simulink model "RocketAirBrake_Simulation"  (R2018b)
settings: Solver=VariableStepAuto  StartTime=0.0  StopTime=30  RelTol=1e-3
undefined symbols (not defined in the file or in its folder): INTAB1, INTAB3, INTAB4
libraries: embdlinuxlib x5, simulink x1
settings Model: Creator=benkl  LastModifiedBy=Alan

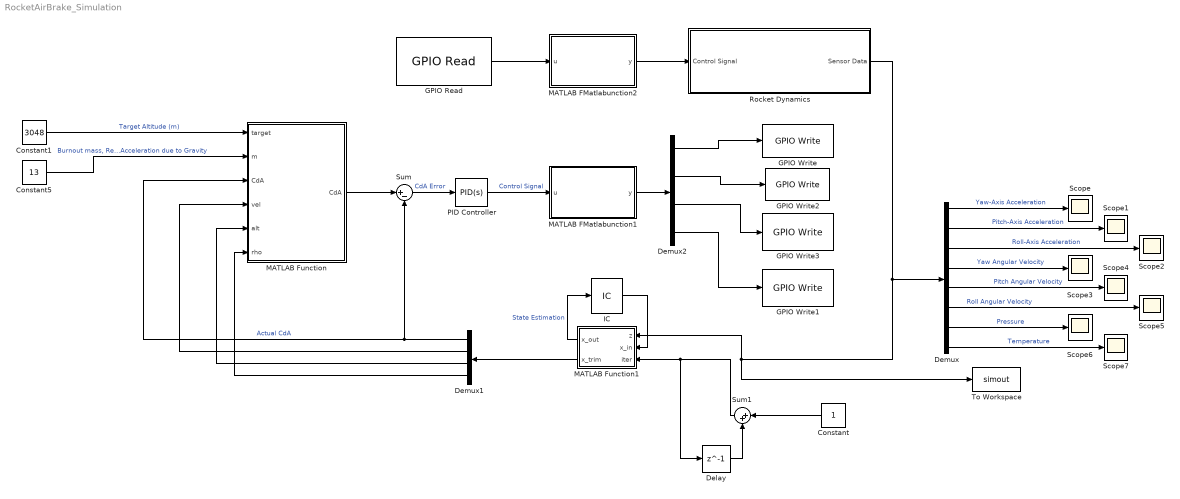
== system RocketAirBrake_Simulation ==
  Constant : Constant
  Constant1 : Constant  Value=3048
  Constant5 : Constant  Value=13
  Delay : Delay  DelayLength=1  InitialCondition=0
  Demux : Demux  Outputs=8
  Demux1 : Demux
  Demux2 : Demux
  GPIO Read : embdlinuxlib/GPIO Read  board=Model B+  gpio=4  internalResistor=Off  sampleTime=0.1  direction=Input  blockPlatform=Raspberry Pi
      settings: SourceProductName=Simulink Support Package for Raspberry Pi Hardware  SourceProductBaseCode=RASPPI
  GPIO Write{,1..3} (4 alike) : embdlinuxlib/GPIO Write  board=Model B+  gpio=17  direction=Output  blockPlatform=Raspberry Pi
      settings: SourceProductName=Simulink Support Package for Raspberry Pi Hardware  SourceProductBaseCode=RASPPI
  IC : InitialCondition  Value=[0;0;0;0;0;0;0;0;0;0;0;0]
  MATLAB FMatlabunction1 : MATLAB Function  TreatAsAtomicUnit=on
  MATLAB FMatlabunction2 : MATLAB Function  TreatAsAtomicUnit=on
  MATLAB Function : MATLAB Function  TreatAsAtomicUnit=on
  MATLAB Function1 : MATLAB Function  TreatAsAtomicUnit=on
  PID Controller : simulink/Continuous/PID Controller  Controller=PID  Form=Parallel  TimeDomain=Continuous-time  SampleTime=-1  IntegratorMethod=Forward Euler  FilterMethod=Forward Euler  ControllerParametersSource=internal  P=1  I=0  D=0  UseFilter=on  N=100  TunerSelectOption=Transfer Function Based (PID Tuner App)  InitialConditionSource=internal  InitialConditionForIntegrator=0  InitialConditionForFilter=0  DifferentiatorICPrevScaledInput=0  ExternalReset=none  TrackingMode=off  Kt=1  LimitOutput=off  UpperSaturationLimit=inf  LowerSaturationLimit=-inf  LinearizeAsGain=on  AntiWindupMode=none  Kb=1  POutMin=[]  POutMax=[]  IOutMin=[]  IOutMax=[]  DOutMin=[]  DOutMax=[]  NOutMin=[]  NOutMax=[]  SumOutMin=[]  SumOutMax=[]  SaturationOutMin=[]  SaturationOutMax=[]  PParamMin=[]  PParamMax=[]  IParamMin=[]  IParamMax=[]  DParamMin=[]  DParamMax=[]  NParamMin=[]  NParamMax=[]  KbParamMin=[]  KbParamMax=[]  KtParamMin=[]  KtParamMax=[]  KbOutMin=[]  KbOutMax=[]  KtOutMin=[]  KtOutMax=[]  IntegratorOutMin=[]  IntegratorOutMax=[]  FilterOutMin=[]  FilterOutMax=[]  SumI1OutMin=[]  SumI1OutMax=[]  SumI2OutMin=[]  SumI2OutMax=[]  SumI3OutMin=[]  SumI3OutMax=[]  SumI4OutMin=[]  SumI4OutMax=[]  SumDOutMin=[]  SumDOutMax=[]  DifferentiatorOutMin=[]  DifferentiatorOutMax=[]  FilterDiffOutCoefMin=[]  FilterDiffOutCoefMax=[]  ReciprocalOutMin=[]  ReciprocalOutMax=[]  SumDenOutMin=[]  SumDenOutMax=[]  SumNumOutMin=[]  SumNumOutMax=[]  DivideOutMin=[]  DivideOutMax=[]  IntegratorContinuousStateAttributes=''  IntegratorStateMustResolveToSignalObject=off  IntegratorRTWStateStorageClass=Auto  FilterContinuousStateAttributes=''  FilterStateMustResolveToSignalObject=off  FilterRTWStateStorageClass=Auto  ParallelPVariant=InternalParameters  IdealPVariant=Disabled  IVariant=InternalParameters  DVariant=InternalParameters  IntegratorVariant=Continuous  SatVariant=Disabled  AWVariant=Passthrough  PCopyVariant=Disabled  TRVariant=Disabled  FdbkBlocksVariant=Forward  IdealPFdbkVariant=Disabled  SatFdbkVariant=Disabled  DerivativeFilterVariant=ContFilter  NVariant=InternalParameters  NCopyVariant=Disabled  FilterICVariant=InternalICsFilter  IntegratorICVariant=InternalICs  ExternalResetVariant=Disabled  TRSumVariant=Passthrough  SumFdbkVariant=Disabled  SumVariant=Sum_PID
  Rocket Dynamics : Subsystem
  Scope{,1..7} (8 alike) : Scope
  Sum : Sum  Inputs=|+-
  Sum1 : Sum  Inputs=|++
  To Workspace : ToWorkspace  VariableName=simout  SaveFormat=Timeseries  SampleTime=-1
  wires:
  Demux/1 -> Scope/1  "Yaw-Axis Acceleration"
  Demux/2 -> Scope1/1  "Pitch-Axis Acceleration"
  Constant1/1 -> MATLAB Function/1(target)  "Target Altitude (m)"
  MATLAB Function/1(CdA) -> Sum/1
  Constant5/1 -> MATLAB Function/2(m)  "Burnout mass, Reference Area,  Acceleration due to Gravity"
  Demux1/1 -> MATLAB Function/3("CdA "), Sum/2  "Actual CdA"
  Demux1/2 -> MATLAB Function/4(vel)
  Demux1/3 -> MATLAB Function/5(alt)
  Demux1/4 -> MATLAB Function/6(rho)
  Sum/1 -> PID Controller/1  "CdA Error"
  Rocket Dynamics/1(Sensor Data) -> To Workspace/1, MATLAB Function1/1(z), Demux/1
  Demux/8 -> Scope7/1  "Temperature"
  Demux/3 -> Scope2/1  "Roll-Axis Acceleration"
  Demux/4 -> Scope3/1  "Yaw Angular Velocity"
  Demux/5 -> Scope4/1  "Pitch Angular Velocity"
  Demux/6 -> Scope5/1  "Roll Angular Velocity"
  Demux/7 -> Scope6/1  "Pressure"
  GPIO Read/1 -> MATLAB FMatlabunction2/1(u)
  MATLAB FMatlabunction2/1(y) -> Rocket Dynamics/1(Control Signal)
  PID Controller/1 -> MATLAB FMatlabunction1/1(u)  "Control Signal"
  MATLAB FMatlabunction1/1(y) -> Demux2/1
  Demux2/4 -> GPIO Write1/1
  Demux2/3 -> GPIO Write3/1
  Demux2/2 -> GPIO Write2/1
  Demux2/1 -> GPIO Write/1
  MATLAB Function1/1(x_out) -> IC/1  "State Estimation"
  MATLAB Function1/2(x_trim) -> Demux1/1
  IC/1 -> MATLAB Function1/2(x_in)
  Constant/1 -> Sum1/1
  Sum1/1 -> Delay/1, MATLAB Function1/3(iter)
  Delay/1 -> Sum1/2

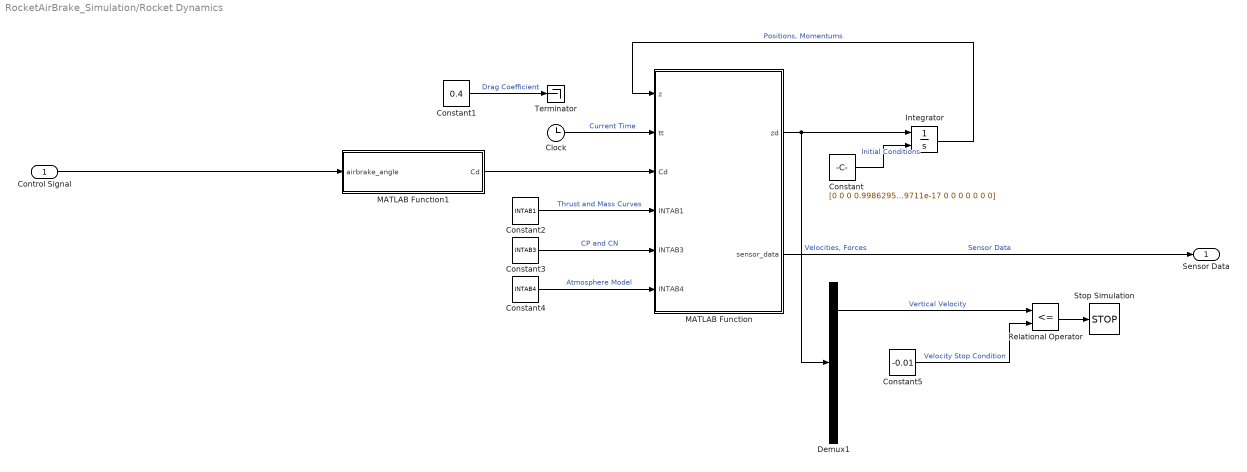
== system RocketAirBrake_Simulation/Rocket Dynamics ==
  Control Signal : Inport
  Clock : Clock
  Constant : Constant  Value="[0\t0\t0\t0.998629534754574\t-0.0523359562429438\t1.92279183879711e-17\t0\t0\t0\t0\t0\t0\t0]"
  Constant1 : Constant  Value=0.4
  Constant2 : Constant  Value=INTAB1  VectorParams1D=off
  Constant3 : Constant  Value=INTAB3  VectorParams1D=off
  Constant4 : Constant  Value=INTAB4  VectorParams1D=off
  Constant5 : Constant  Value=-0.01
  Demux1 : Demux  Outputs=13
  Integrator : Integrator  InitialConditionSource=external
  MATLAB Function : MATLAB Function  TreatAsAtomicUnit=on
  MATLAB Function1 : MATLAB Function  TreatAsAtomicUnit=on
  Relational Operator : RelationalOperator  Operator=<=  OutDataTypeStr=boolean  RndMeth=Simplest
  Stop Simulation : Stop
  Terminator : Terminator
  Sensor Data : Outport
  wires:
  Clock/1 -> MATLAB Function/2(tt)  "Current Time"
  Integrator/1 -> MATLAB Function/1(z)  "Positions, Momentums"
  Constant4/1 -> MATLAB Function/6(INTAB4)  "Atmosphere Model"
  Demux1/3 -> Relational Operator/1  "Vertical Velocity"
  MATLAB Function/1(zd) -> Demux1/1, Integrator/1  "Velocities, Forces"
  Relational Operator/1 -> Stop Simulation/1
  Constant5/1 -> Relational Operator/2  "Velocity Stop Condition"
  Constant3/1 -> MATLAB Function/5(INTAB3)  "CP and CN"
  Constant2/1 -> MATLAB Function/4(INTAB1)  "Thrust and Mass Curves"
  Constant/1 -> Integrator/2  "Initial Conditions"
  MATLAB Function/2(sensor_data) -> Sensor Data/1  "Sensor Data"
  Control Signal/1 -> MATLAB Function1/1(airbrake_angle)
  MATLAB Function1/1(Cd) -> MATLAB Function/3(Cd)
  Constant1/1 -> Terminator/1  "Drag Coefficient"

== matlab function RocketAirBrake_Simulation/MATLAB Function ==
  data: target input; m input; CdA output; CdA input; vel input; alt input; rho input
function CdA  = drag_predictor(target, m, CdA, vel, alt, rho)
%DRAG_PREDICTOR calculates the optimal drag coefficient based on current state

in.alt = alt; % [m] rocket's current altitude
in.vel = vel; % [m/s] rocket's current velocity
in.rho = rho; % [kg/m^3] density of air
in.m = m; % [kg] mass of rocket after burnout

CdA_opt = secant(@apogeeerror, CdA, in); % Might want to use a more robust solver in the future

if CdA_opt > 0.001 && CdA_opt < 0.01 % Set upper and lower bounds on CdA (m^2)
    CdA = CdA_opt;
end % Otherwise keep estimated term for CdA

    function [x] = secant(fun, x1, in)
    %SECANT is a zero-finding function based on the secant method
    %   'fun' is the function handle for which the zero is desired
    %   'x1' is the initial guess
    %   'in' is a struct containing any additional inputs 'fun' might require
    %   'x' is the value of the zero
        x_eps = x1*0.005; % Set the tolerance to be 0.5% of initial guess
        x2 = x1-x1*0.01; % Set a second point 1% away from the original guess
        F1 = fun(x1, in); % Evaluate function at x1
        F2 = fun(x2, in); % Evaluate function at x2
        kk = 1; % Set up counter
        kk_max = 100;
        while abs(x2-x1)>=x_eps && kk<kk_max % While error is too large and counter is less than max
            x3 = x2 - F2*(x2-x1)/(F2-F1);
            x1 = x2; % Move everything forward
            x2 = x3;
            F1 = F2;
            F2 = fun(x2, in);
            kk = kk+1;
        end
        x = x2;
    end

    function apogee = apogeeerror(CdA, in) % Finds the difference between the estimated and actual apogee
        apogee = in.alt + in.m/(CdA*in.rho) * log( CdA*in.rho/(2*in.m*9.81) * in.vel^2 + 1 ) - target;
    end

end

== matlab function RocketAirBrake_Simulation/Rocket Dynamics/MATLAB Function ==
  data: z input; tt input; zd output; Cd input; INTAB1 input; INTAB3 input; INTAB4 input; sensor_data output
function [zd,sensor_data]=blastoff6dof(z,tt,Cd,INTAB1,INTAB3,INTAB4)

% Constants **************************************************************
RL=4.3; % Launch rail length
Ar=0.010751315458748; % Rocket aerodynamic reference area


% Unpack z ***************************************************************
xn=z(1); % Postion vector
yn=z(2); % "
zn=z(3); % "
s=z(4); % Quaternion scalar
vx=z(5); % Quaternion vector
vy=z(6); % "
vz=z(7); % "
Px=z(8); % Translational momentum vector
Py=z(9); % "
Pz=z(10); % "
Ltheta=z(11); % Rotational momentum vector
Lphi=z(12); % "
Lpsi=z(13); % "

xt=[xn;yn;zn]; % Rocket position vector
qt=[s vx vy vz]; % Rocket quaternion
Pt=[Px;Py;Pz]; % Rocket translational momentum vector
Lt=[Ltheta;Lphi;Lpsi]; % Rocket rotational momentum vector


% Gravity ****************************************************************
g=6.6742E-11*5.9742E24/(6378100+zn)^2;


% EXTRACT DATA FROM INPUT TABLES 1, 3, and 4 *****************************
% INTAB1 *****************************************************************
t=INTAB1(:,1); % Get time data from input table
if tt<=t(1)
    Ti=INTAB1(1,2);
    Mi=INTAB1(1,3);
    Ixxi=INTAB1(1,4);
    Iyyi=INTAB1(1,5);
    Izzi=INTAB1(1,6);
    Ixyi=INTAB1(1,7);
    Ixzi=INTAB1(1,8);
    Iyzi=INTAB1(1,9);
    Xcmi=INTAB1(1,10);
    Cda1=INTAB1(1,11);
elseif tt<t(end) && tt>=t(1) % If time is within bounds of array
    Ti=interp1(t,INTAB1(:,2),tt); % Thrust-time data
    Mi=interp1(t,INTAB1(:,3),tt); % Mass-time data
    Ixxi=interp1(t,INTAB1(:,4),tt); % Moments of inertia-time data
    Iyyi=interp1(t,INTAB1(:,5),tt); % "
    Izzi=interp1(t,INTAB1(:,6),tt); % "
    Ixyi=interp1(t,INTAB1(:,7),tt); % Products of inertia-time data
    Ixzi=interp1(t,INTAB1(:,8),tt); % "
    Iyzi=interp1(t,INTAB1(:,9),tt); % "
    Xcmi=interp1(t,INTAB1(:,10),tt); % Center of mass-time data
    Cda1=interp1(t,INTAB1(:,11),tt); % Thrust damping moment coefficient
else
    Ti=INTAB1(end,2);
    Mi=INTAB1(end,3);
    Ixxi=INTAB1(end,4);
    Iyyi=INTAB1(end,5);
    Izzi=INTAB1(end,6);
    Ixyi=INTAB1(end,7);
    Ixzi=INTAB1(end,8);
    Iyzi=INTAB1(end,9);
    Xcmi=INTAB1(end,10);
    Cda1=INTAB1(end,11);
end
Ibody=[Ixxi Ixyi Ixzi;Ixyi Iyyi Iyzi;Ixzi Iyzi Izzi]; % Inertia tensor

% INTAB3 *****************************************************************
Cn=INTAB3(1);
Cp=INTAB3(2);

% INTAB4 *****************************************************************
ztb=INTAB4(:,1); %Get altitude data from input table
if zn<ztb(end) && zn>=ztb(1)
    Wxi=interp1(ztb,INTAB4(:,2),zn);%Wind velocity vector
    Wyi=interp1(ztb,INTAB4(:,3),zn);%"
    Wzi=interp1(ztb,INTAB4(:,4),zn);%"
    
    rho=interp1(ztb,INTAB4(:,5),zn);%Atmospheric density
    temp=interp1(ztb,INTAB4(:,6),zn);%Atmospheric Temperature
    Pressure = 287*rho*temp;%Atmospheric Pressure
else % If outside of table bounds
    Wxi=INTAB4(end,2);%Wind velocity vector
    Wyi=INTAB4(end,3);%"
    Wzi=INTAB4(end,4);%"
    
    temp=(-131.21+(0.00299*zn))+273.15; % Random atmosphere model???
    Pressure=0.002488*(temp/216.6)^-11.388;
    rho=Pressure/287*temp;
end


% Rocket Velocity Calculations *******************************************
if vectormag(xt)<=RL % While vehicle is still on the launch rail
    Wt=[0;0;0];
else
    Wt=[Wxi;Wyi;Wzi]; % Wind vector
end
Ut=Pt./Mi; % Rocket earth relative velocity vector
Vt=Ut+Wt; % Rocket atmosphere relative velocity vector


% Rocket orientation calculations ****************************************
qt=vectornorm(qt); % Normalise quaternion
s=qt(1); % Quaternion scalar part only
vt=[qt(2);qt(3);qt(4)]; % Quaternion vector part only
Rt=quaternion_to_matrix(qt); % Transform quaternion to rotation matrix
RA=Rt*[0;0;1]; % Roll axis vector


% Center of pressure velocity calculations *******************************
Xbar=Cp-Xcmi; % Moment arm
Xbart=-Xbar*RA; % Moment arm vector

It = Rt*Ibody*Rt'; % Inertia tensor in global coordinates
omegat=It\Lt; % Angular velocity vector

Vcpt=Vt+cross(omegat, Xbart); % Velocity vector of center of pressure
Vcptmag=vectormag(Vcpt); % Magnitude of velocity of center of pressure
Vcptnorm=vectornorm(Vcpt); % Direction of velocity of center of pressure

if Vcptmag==0 % Set angle of attack to zero if not moving
    alphacp=0;
else
    dprod=dot(Vcptnorm,RA); % Dot product of velocity and rocket axis
    if dprod>1
        dprod=1;
    end
    alphacp=acos(dprod); % Angle of attack
end


% Force vector calculations **********************************************
FA=Cd*0.5*rho*(Vcptmag^2)*Ar*cos(alphacp); % Calculate axial aerodynamic force
FAt=FA*-RA; % Axial drag vector

FNcp=Cn*alphacp*0.5*rho*(Vcptmag^2)*Ar*sin(alphacp); % Calculate normal aerodynamic force
momaxcp=cross(RA,Vcptnorm); % axis of pitching motion
momaxcp=vectornorm(momaxcp);
FNn=cross(RA,momaxcp);
FNn=vectornorm(FNn); % Direction of normal force
FNt=FNcp*FNn; % Normal force vector

Tt=Ti*RA; % Thrust Vector

mg=Mi*g; % Gravity

% Torque vector calculations *********************************************
Tqf=(FNcp*Xbar)*momaxcp; % Aerodynamic torque due to normal force
Tqm=-Cda1*omegat; % Thrust damping torque
% Tqm=(-Cda1*omega)*omegaax2; % Thrust damping torque
Tqt=Tqf+Tqm; % Total torque on rocket


% Output calculations ****************************************************
% Calculate position derivatives (velocities relative to earth)
xdot=Ut(1);
ydot=Ut(2);
zdot=Ut(3);

% Calculate quaternion derivative
sdot=(-dot(omegat,vt))*0.5;
vtdot=((s*omegat)+(cross(omegat,vt)))*0.5;
vxdot=vtdot(1);
vydot=vtdot(2);
vzdot=vtdot(3);

% Calculate translational momentum derivatives (forces)
if Ti<=mg && zn<0.1 % If thrust is smaller than gravity and flight just began
    Fx=0;
    Fy=0;
    Fz=0;
else
    Fx=Tt(1)+FAt(1)+FNt(1); % X Force vector component
    Fy=Tt(2)+FAt(2)+FNt(2); % Y Force vector component
    Fz=Tt(3)+FAt(3)+FNt(3)-mg; % Z Force vector component
end

% Calculate rotational momentum derivatives (torques)
if vectormag(xt)<=RL % While still on launch rail
    Ttheta=0;
    Tphi=0;
    Tpsi=0;
else
    Ttheta=Tqt(1); % Torque vector
    Tphi=Tqt(2); %"
    Tpsi=Tqt(3); %"
end

%ODE output
zd=zeros(13,1);
zd(1)=xdot;
zd(2)=ydot;
zd(3)=zdot;
zd(4)=sdot;
zd(5)=vxdot;
zd(6)=vydot;
zd(7)=vzdot;
zd(8)=Fx;
zd(9)=Fy;
zd(10)=Fz;
zd(11)=Ttheta;
zd(12)=Tphi;
zd(13)=Tpsi;

% Sensor output **********************************************************
Ft = [Fx;Fy;Fz]; % Vector of forces
Fr = Rt'*Ft; % Rotate forces to align with rocket axis
a = Fr./Mi; % Convert forces to accelerations
omegar = Rt'*omegat; % Rotate angular velocities to align with rocket axis

sensor_data=zeros(8,1);
sensor_data(1) = a(1); % Yaw-direction acceleration
sensor_data(2) = a(2); % Pitch-direction acceleration
sensor_data(3) = a(3); % Roll-direction acceleration
sensor_data(4) = omegar(1); % Yaw-direction angular velocity
sensor_data(5) = omegar(2); % Pitch-direction angular velocity
sensor_data(6) = omegar(3); % Roll-direction angular velocity
sensor_data(7) = Pressure; % Atmospheric pressure
sensor_data(8) = temp; % Atmospheric temperature

end

== matlab function RocketAirBrake_Simulation/Rocket Dynamics/MATLAB Function1 ==
  data: airbrake_angle input; Cd output
function Cd = dragTF(airbrake_angle)

%%%%%%%%%%%%%% REPLACE THIS WITH BETTER MODEL BASED ON CFD %%%%%%%%%%%%%%%%
% Also add mach number dependency

Cd_rocket = 0.4; % Coefficient of drag of rocket
A_ref = 0.010751315458748; % [m^2] rocket reference area
Cd_flat_plate = 1.28; % https://www.grc.nasa.gov/www/k-12/airplane/shaped.html
TF = 3.888e-3; % Linear fit of area to angle from Solidworks data

A_flat_plate = TF*airbrake_angle; % Calculate exposed area
Cd = Cd_rocket + Cd_flat_plate*A_flat_plate/A_ref; % Calculate Drag Coefficient

== matlab function RocketAirBrake_Simulation/MATLAB Function1 ==
  data: z input; x_out output; x_in input; iter input; x_trim output
function [x_out,x_trim] = fcn(z,x_in,iter)
%constants and data
Ax = z(1);
Ay = z(2);
Az = z(3);
psi_dot = z(4);
theta_dot = z(5);
phi_dot = z(6);
Pr = z(7);

g = 9.81;
Ix = 2.1638;
Iy = 2.1638;
Iz = 0.0016;
m = 15.7210;

L = -0.0065;
ho = 1200;
To = 287;
Po = 87500;
rate = 0.001;
Rconst = 287.058;

psi = zeros(1,size);
theta = zeros(1,size);
phi = zeros(1,size);

%Kalman Filter initialization
Rot = eye(3);
Q = 100.*eye(14);
R = 5;
P = 100.*eye(14);
A = zeros(14);
H = [0,1,0,0,0,0,0,0,0,0,0,0,0,0;
     0,0,0,1,0,0,0,0,0,0,0,0,0,0;
     0,0,0,0,0,1,0,0,0,0,0,0,0,0;
     0,0,0,0,0,0,0,1,0,0,0,0,0,0;
     0,0,0,0,0,0,0,0,0,1,0,0,0,0;
     0,0,0,0,0,0,0,0,0,0,0,1,0,0];
 
%  x_nom = [body_xyz(1,:);        
%           body_vxyz(1,:);
%           body_xyz(2,:);
%           body_vxyz(2,:);
%           body_xyz(3,:)+1200;
%           body_vxyz(3,:);
%           psi;
%           psi_dot';
%           theta;
%           theta_dot';
%           phi;
%           phi_dot';
%           Cd'
%           Ar*ones(1,size)];
      
   
    psi_P = x_in(7) + rate*psi_dot;
    theta_P = x_in(9) + rate*theta_dot;
    phi_P = x_in(11) + rate*phi_dot;
    
    Rot(1,1) = cosd(phi_P(index))*cosd(theta_P(index));
    Rot(1,2) = -sind(phi_P(index))*cosd(psi_P(index))+cosd(phi_P(index))*sind(theta_P(index))*sind(psi_P(index));
    Rot(1,3) = sind(phi_P(index))*sind(psi_P(index))+cosd(phi_P(index))*sind(theta_P(index))*cosd(psi_P(index));
    Rot(2,1) = sind(phi_P(index))*cosd(theta_P(index));
    Rot(2,2) = cosd(phi_P(index))*cosd(psi_P(index))+sind(phi_P(index))*sind(theta_P(index))*sind(psi_P(index));
    Rot(2,3) = -cosd(phi_P(index))*sind(psi_P(index))+sind(phi_P(index))*sind(theta_P(index))*cosd(psi_P(index));
    Rot(3,1) = -sind(theta_P(index));
    Rot(3,2) = cosd(theta_P(index))*sind(psi_P(index));
    Rot(3,3) = cosd(theta_P(index))*cosd(psi_P(index));
    
    Vx_P = x_in(2) + rate*Ax;
    Vy_P = x_in(4) + rate*Ay;
    Vz_P = x_in(6) + rate*Az;
            
    T = To*((Pr/Po)^(L*Rconst/g));
    Z = (Rconst*T/g)*log(Pr/Po);
    z = rot*[0;0;Z];
    rho_c = Pr/(Rconst*T);
     y = [Vx_P;Vy_P;z;Vz_P;psi_dot;theta_dot;phi_dot];  
   
    
    
    k = P*H'/(H*P*H' + R);
    P = (eye(14)-k*H)*P;
%   P = (eye(14) - k*H)*P*(eye(14)-k*H)' + (k*R*k')/gamma;
    x = x_in + k*(y-H*x_in);
   
    A(1,2) = 1;
    A(2,7) = -g*(cosd(x_nom(7,index))*sind(x_nom(11,index))+sind(x_nom(7,index))*sind(x_nom(9,index))*cosd(x_nom(11,index)));
    A(2,9) = g*cosd(x_nom(7,index))*cosd(x_nom(9,index))*cosd(x_nom(11,index));
    A(2,11) = -g*(sind(x_nom(7,index))*cosd(x_nom(11,index))+cosd(x_nom(7,index))*sind(x_nom(9,index))*cosd(x_nom(11,index)));
    A(3,4) = 1;
    A(4,7) = g*(cosd(x_nom(7,index))*cosd(x_nom(11,index))+sind(x_nom(7,index))*sind(x_nom(9,index))*sind(x_nom(11,index)));
    A(4,9) = -g*cosd(x_nom(7,index))*cosd(x_nom(9,index))*sind(x_nom(11,index));
    A(4,11) = -g*(sind(x_nom(7,index))*sind(x_nom(11,index))+cosd(x_nom(7,index))*sind(x_nom(9,index))*cosd(x_nom(11,index)));
    A(5,6) = 1;
    A(6,6) = -x_nom(13,index)*x_nom(14,index)*rho_c(index)*x_nom(6,index)/m;
    A(6,7) = g*sind(x_nom(7,index))*cosd(x_nom(9,index));
    A(6,9) = g*cosd(x_nom(7,index))*sind(x_nom(9,index));
    A(6,13) = x_nom(14,index)*rho_c(index)*(x_nom(6,index)^2)/(2*m);
    A(6,14) = x_nom(13,index)*rho_c(index)*(x_nom(6,index)^2)/(2*m);
    A(7,8) = 1;
    A(8,10) = ((Iy-Iz)/Ix)*x_nom(12,index);
    A(8,12) = ((Iy-Iz)/Ix)*x_nom(10,index);
    A(9,10) = 1;
    A(10,8) = ((Iz-Ix)/Iy)*x_nom(12,index);
    A(10,12) = ((Iy-Iz)/Ix)*x_nom(8,index);
    A(11,12) = 1;
    A(12,8) = ((Ix-Iy)/Iz)*x_nom(10,index);
    A(12,10) = ((Ix-Iy)/Iz)*x_nom(8,index);
    A(13,13) = 1;
    A(14,14) = 1;
       
    P = A*P*A'+Q;
    x = A*x;
    
%     x_out(:,index) = x + x_nom(:,index);
%     Cd_hat(index)  = x_out(13,index);
%     Ar_hat(index) = x_out(14,index);
%     temp       = Rot\[x_out(1,index);x_out(3,index);x_out(5,index)];
%     Z_hat(index)   = temp(3);
%     temp       = Rot\[x_out(2,index);x_out(4,index);x_out(6,index)];       
%     V_hat(index)   = temp(3);
    
% Ar = Ar*ones(1,size);
% plot(t,Cd_hat,t,Cd);
% legend("Estimated Drag Coefficient","Actual Drag Coefficient");
% xlabel("Time [s]");
% ylabel("Drag Coefficient");
% 
% figure()
% plot(t,rho,t,rho_c);
% legend("Actual Density","Calculated Density");
% xlabel("Time [s]");
% ylabel("Air Density");
% 
% figure()
% plot(t,Z_hat,t,Z_Act);
% legend("Estimated Altitude","Actual Altitude");
% xlabel("Time [s]");
% ylabel("Altitude");
% 
% figure()
% plot(t,V_hat,t,V_Act);
% legend("Estimated Velocity","Actual Velocity");
% xlabel("Time [s]");
% ylabel("Vertical Velocity");
% 
% figure()
% plot(t,Ar_hat,t,Ar);
% legend("Estimated Area","Actual Area");
% xlabel("Time [s]");
% ylabel("Area");

y = z;

== matlab function RocketAirBrake_Simulation/MATLAB FMatlabunction2 ==
  data: u input; y output
function y = Steps_to_Angle_TF(u)
%#codegen

y = u;

== matlab function RocketAirBrake_Simulation/MATLAB FMatlabunction1 ==
  data: u input; y output
function y  = Error_To_Steps(u)
%#codegen

y = u;
